simulink model "SimulacionTanqueControlado"  (R2020a)
settings: Solver=VariableStepAuto  StartTime=0.0  StopTime=tsim  RelTol=1e-3
values from neighbouring files (symbols this model uses):
  alpha = 1    [ParametrosTanque.m]
  Area = 1    [ParametrosTanque.m]
  K1 = 1    [ParametrosTanque.m]
  K2 = K1    (= 1)    [ParametrosTanque.m]
  Kp = .01    (= 0.01)    [ParametrosTanque.m]
  T1 = 90    [ParametrosTanque.m]
  T2 = 10    [ParametrosTanque.m]
  tau1 = 5    [ParametrosTanque.m]
  tau2 = 4    [ParametrosTanque.m]
  tdelay1 = 2 * tmuestra    [ParametrosTanque.m]
  tdelay2 = tmuestra    [ParametrosTanque.m]
  tdelayQ = tmuestra    [ParametrosTanque.m]
  Te = 45    [ParametrosTanque.m]
undefined symbols (not defined in the file or in its folder): ControlBorrosoIncremental, FuzzySetQ, FuzzySetT, Qi, Ti, tmuestra, Ui, Yr
settings Model: Creator=pablo  LastModifiedBy=pablo
settings DataIOCC: SaveOutput=off  SignalLogging=off  DSMLogging=off  SaveTime=off  ReturnWorkspaceOutputs=off
settings DebuggingCC: UnderSpecifiedDimensionMsg=warning  ArithmeticOperatorsInVariantConditions=warning
settings SFSimCC: CustomCodeUndefinedFunction=UseInterfaceOnly

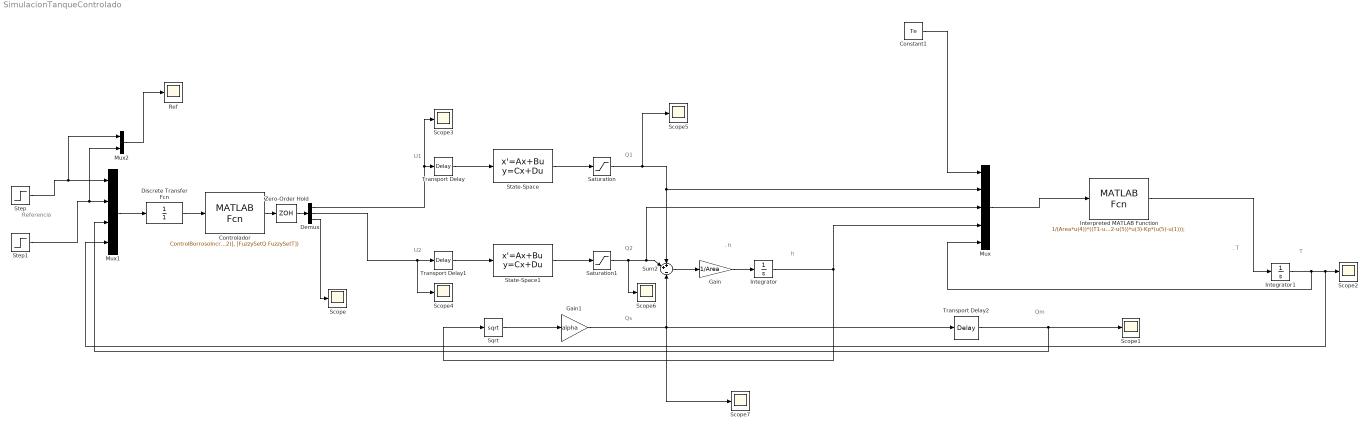
== system SimulacionTanqueControlado ==
  note: Referencia
  note: Qm
  note: .
      | T
  note: T
  note: h
  note: .
      |  h
  note: Qs
  note: Q1
  note: U1
  note: Q2
  note: U2
  Constant1 : Constant  Value=Te
  Controlador : MATLABFcn  MATLABFcn=ControlBorrosoIncremental([u(1); u(2)], [u(3); u(4)], [0 4; 0 4], [u(1); u(2)], [FuzzySetQ FuzzySetT])  OutputDimensions=4
  Demux : Demux  Outputs=[1 1 2]
  Discrete Transfer Fcn : DiscreteTransferFcn  Numerator=1  Denominator=1  SampleTime=tmuestra
  Gain : Gain  Gain=1/Area
  Gain1 : Gain  Gain=alpha
  Integrator : Integrator  InitialCondition=(Qi/alpha)^2  LimitOutput=on  LowerSaturationLimit=0
  Integrator1 : Integrator  InitialCondition=Ti  LowerSaturationLimit=0
  Interpreted MATLAB Function : MATLABFcn  MATLABFcn=1/(Area*u(4))*((T1-u(5))*u(2)+(T2-u(5))*u(3)-Kp*(u(5)-u(1)));  OutputDimensions=1
  Mux : Mux  Inputs=5
  Mux1 : Mux
  Mux2 : Mux  Inputs=2
  Ref : Scope
  Saturation : Saturate  UpperLimit=inf  LowerLimit=0
  Saturation1 : Saturate  UpperLimit=inf  LowerLimit=0
  Scope{,1..7} (8 alike) : Scope
  Sqrt : Sqrt  SaturateOnIntegerOverflow=on
  State-Space : StateSpace  A=-1/tau1  B=K1/tau1  D=0  InitialCondition=Ui(1)
  State-Space1 : StateSpace  A=-1/tau2  B=K2/tau2  D=0  InitialCondition=Ui(2)
  Step : Step  Time=10  Before=Qi  After=Yr(1)  SampleTime=tmuestra
  Step1 : Step  Time=10  Before=Ti  After=Yr(2)  SampleTime=tmuestra
  Sum2 : Sum  Inputs=++|-
  Transport Delay : TransportDelay  DelayTime=tdelay1  InitialOutput=Ui(1)
  Transport Delay1 : TransportDelay  DelayTime=tdelay2  InitialOutput=Ui(2)
  Transport Delay2 : TransportDelay  DelayTime=tdelayQ  InitialOutput=Qi
  Zero-Order Hold : ZeroOrderHold  SampleTime=tmuestra
  wires:
  Demux/1 -> Scope3/1, Transport Delay/1
  Transport Delay/1 -> State-Space/1
  State-Space/1 -> Saturation/1
  Transport Delay1/1 -> State-Space1/1
  State-Space1/1 -> Saturation1/1
  Demux/2 -> Scope4/1, Transport Delay1/1
  Sum2/1 -> Gain/1
  Gain1/1 -> Scope7/1, Sum2/3, Transport Delay2/1
  Sqrt/1 -> Gain1/1
  Gain/1 -> Integrator/1
  Integrator/1 -> Sqrt/1, Mux/4
  Saturation/1 -> Scope5/1, Mux/2, Sum2/1
  Saturation1/1 -> Scope6/1, Mux/3, Sum2/2
  Constant1/1 -> Mux/1
  Integrator1/1 -> Mux/5, Mux1/4, Scope2/1
  Transport Delay2/1 -> Mux1/3, Scope1/1
  Step/1 -> Mux2/1, Mux1/1
  Step1/1 -> Mux2/2, Mux1/2
  Demux/3 -> Scope/1
  Mux1/1 -> Discrete Transfer Fcn/1
  Discrete Transfer Fcn/1 -> Controlador/1
  Controlador/1 -> Zero-Order Hold/1
  Zero-Order Hold/1 -> Demux/1
  Interpreted MATLAB Function/1 -> Integrator1/1
  Mux/1 -> Interpreted MATLAB Function/1
  Mux2/1 -> Ref/1
